simulink model "PT2Regler"  (R2021b)
settings: Solver=VariableStepAuto  StartTime=0.0  StopTime=10.0  RelTol=1e-3
model workspace (MAT data in the model file):
  D = Simulink.Parameter
  D.Value = [0 0.2 1]
  D.DataType = 'auto'
  D.Complexity = 'real'
  D.Dimensions = [1 3]
  D1 = Simulink.Parameter
  D1.Value = [0 0.25 1]
  D1.DataType = 'auto'
  D1.Complexity = 'real'
  D1.Dimensions = [1 3]
  Kr = Simulink.Parameter
  Kr.Value = 0.5
  Kr.DataType = 'auto'
  Kr.Complexity = 'real'
  Kr.Dimensions = [1 1]
  N = Simulink.Parameter
  N.Value = [0.9 1]
  N.DataType = 'auto'
  N.Complexity = 'real'
  N.Dimensions = [1 2]
  N1 = Simulink.Parameter
  N1.Value = [0.5 1]
  N1.DataType = 'auto'
  N1.Complexity = 'real'
  N1.Dimensions = [1 2]
settings Model: ParameterArgumentNames=Kr,N,D,N1,D1  Creator=Hoorsana  LastModifiedBy=Hoorsana

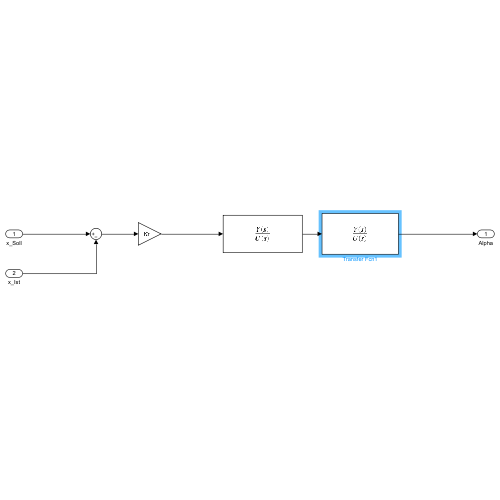
[thumbnail: Simulink's stored preview of the top-level diagram]
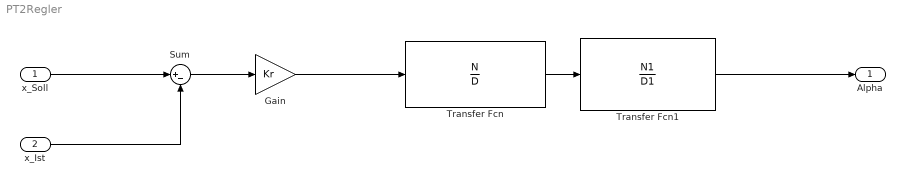
== system PT2Regler ==
  x_Soll : Inport
  x_Ist : Inport  Port=2
  Gain : Gain  Gain=Kr
  Sum : Sum  Inputs=|+-
  Transfer Fcn : TransferFcn  Numerator=N  Denominator=D
  Transfer Fcn1 : TransferFcn  Numerator=N1  Denominator=D1
  Alpha : Outport
  wires:
  Transfer Fcn/1 -> Transfer Fcn1/1
  Transfer Fcn1/1 -> Alpha/1
  Sum/1 -> Gain/1
  Gain/1 -> Transfer Fcn/1
  x_Ist/1 -> Sum/2
  x_Soll/1 -> Sum/1
